simulink model "Trofazni_mosni_punoupravljivi_tiristorski_ispravljac"  (R2014b)
settings: Solver=ode5  StartTime=0.0  StopTime=1  FixedStep=Tsim  MaxStep=Tsim  RelTol=1e-3
values from neighbouring files (symbols this model uses):
  alfa = 60    [ParametriMfajl.m]
  f = 50    [ParametriMfajl.m]
  L = 10e-3    (= 0.01)    [ParametriMfajl.m]
  R = 10    [ParametriMfajl.m]
  Vmax = 220*sqrt(2)    [ParametriMfajl.m]
libraries: powerlib x20, powerlib_meascontrol x1
settings Model: Creator=Korisnik  LastModifiedBy=Zorana

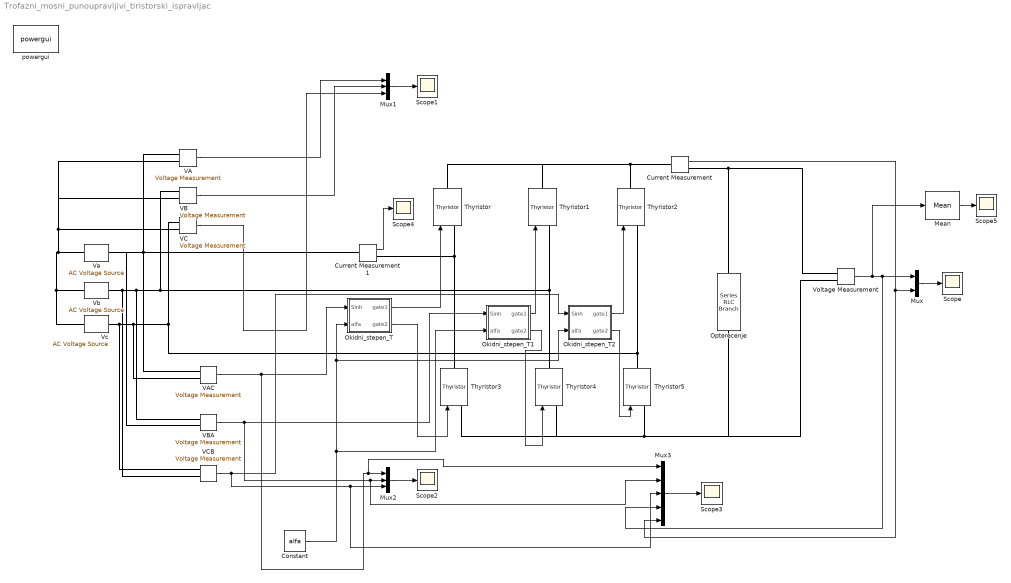
== system Trofazni_mosni_punoupravljivi_tiristorski_ispravljac ==
  Constant : Constant  Value=alfa
  Current Measurement : powerlib/Measurements/Current Measurement  PhasorSimulation=off  OutputType=Complex  PSBequivalent=0
  Current Measurement1 : powerlib/Measurements/Current Measurement  PhasorSimulation=off  OutputType=Complex  PSBequivalent=0
  Mean : powerlib_meascontrol/Measurements/Mean  Freq=f  Vinit=0  Ts=0
  Mux : Mux  Inputs=2
  Mux1 : Mux  Inputs=3
  Mux2 : Mux  Inputs=3
  Mux3 : Mux  Inputs=5
  Okidni_stepen_T : Subsystem
  Okidni_stepen_T1 : Subsystem
  Okidni_stepen_T2 : Subsystem
  Opterecenje : powerlib/Elements/Series RLC Branch  LConnTagsString=__new0  RConnTagsString=__new0  BranchType=RL  Resistance=R  Inductance=L*100  SetiL0=off  InitialCurrent=0  Capacitance=1e-6  Setx0=off  InitialVoltage=0  Measurements=None
  Scope{,1..5} (6 alike) : Scope
      Scope settings: YMin=-300  YMax=300
      Scope2 settings: SaveName=ScopeData2
      Scope3 settings: SaveName=ScopeData3
      Scope4 settings: SaveName=ScopeData4
      Scope5 settings: YMin=-300  YMax=300  SaveName=ScopeData5
  Thyristor{,1..5} (6 alike) : powerlib/Power Electronics/Thyristor  Ron=1e-6  Lon=0  Vf=0  IC=0  Rs=500  Cs=250e-9  Measurements=off
  VA : powerlib/Measurements/Voltage Measurement  PhasorSimulation=off  OutputType=Complex  PSBequivalent=0
  VAC : powerlib/Measurements/Voltage Measurement  PhasorSimulation=off  OutputType=Complex  PSBequivalent=0
  VB : powerlib/Measurements/Voltage Measurement  PhasorSimulation=off  OutputType=Complex  PSBequivalent=0
  VBA : powerlib/Measurements/Voltage Measurement  PhasorSimulation=off  OutputType=Complex  PSBequivalent=0
  VC : powerlib/Measurements/Voltage Measurement  PhasorSimulation=off  OutputType=Complex  PSBequivalent=0
  VCB : powerlib/Measurements/Voltage Measurement  PhasorSimulation=off  OutputType=Complex  PSBequivalent=0
  Va : powerlib/Electrical Sources/AC Voltage Source  Amplitude=Vmax  Phase=0  Frequency=f  SampleTime=0  Measurements=None
  Vb : powerlib/Electrical Sources/AC Voltage Source  Amplitude=Vmax  Phase=-120  Frequency=f  SampleTime=0  Measurements=None
  Vc : powerlib/Electrical Sources/AC Voltage Source  Amplitude=Vmax  Phase=-240  Frequency=f  SampleTime=0  Measurements=None
  Voltage Measurement : powerlib/Measurements/Voltage Measurement  PhasorSimulation=off  OutputType=Complex  PSBequivalent=0
  powergui : powerlib/powergui  Priority=1  SimulationMode=Continuous  SolverType=Tustin/Backward Euler (TBE)  SampleTime=50e-6  frequency=60  SPID=off  DisableSnubberDevices=off  DisableRonSwitches=off  DisableVfSwitches=off  SwTol=0  DisplayEquations=off  Interpol=off  methode=off  Ts=100  frequencyindice=50  Pbase=100e6  ErrMax=1e-4  Iterations=50  UnitsV=kV  UnitsW=MW  FunctionMessages=off  echomessages=off  HookPort=off  EnableUseOfTLC=off  x0status=blocks  RestoreLinks=warning  ResistiveCurrentMeasurement=off  Frange=[0:2:500]  Ylog=off  Xlog=on  ShowGrid=off  save=off  variable=ZData  structure=0  ZoomFFT=off  StartTime=0.0  cycles=1  DisplayStyle=1  fundamental=60  FreqAxis=off  MaxFrequency=1000  frequencyindicesteady=1  RmsSteady=1  display=off
  wires:
  Voltage Measurement/1 -> Mean/1, Mux/1, Mux3/4
  Mux/1 -> Scope/1
  Mux1/1 -> Scope1/1
  VA/1 -> Mux1/1
  VB/1 -> Mux1/2
  VC/1 -> Mux1/3
  Mux2/1 -> Scope2/1
  Current Measurement/1 -> Mux3/5, Mux/2
  Mux3/1 -> Scope3/1
  Current Measurement1/1 -> Scope4/1
  Mean/1 -> Scope5/1
  VAC/1 -> Mux3/1, Mux2/1, Okidni_stepen_T/1(Sinh)
  Okidni_stepen_T/1(gate1) -> Thyristor/1
  Okidni_stepen_T/2(gate2) -> Thyristor3/1
  Constant/1 -> Okidni_stepen_T2/2(alfa), Okidni_stepen_T/2(alfa), Okidni_stepen_T1/2(alfa)
  VBA/1 -> Mux3/2, Mux2/2, Okidni_stepen_T1/1(Sinh)
  Okidni_stepen_T1/1(gate1) -> Thyristor1/1
  Okidni_stepen_T1/2(gate2) -> Thyristor4/1
  VCB/1 -> Mux3/3, Mux2/3, Okidni_stepen_T2/1(Sinh)
  Okidni_stepen_T2/1(gate1) -> Thyristor2/1
  Okidni_stepen_T2/2(gate2) -> Thyristor5/1
  connections:
  Current Measurement1/RConn1 -- Thyristor/LConn1 -- Thyristor3/RConn1
  Vb/RConn1 -- VCB/LConn2 -- VBA/LConn1 -- VB/LConn1 -- Thyristor1/LConn1 -- Thyristor4/RConn1
  Vc/RConn1 -- VCB/LConn1 -- VAC/LConn2 -- VC/LConn1 -- Thyristor2/LConn1 -- Thyristor5/RConn1
  Thyristor3/LConn1 -- Thyristor4/LConn1 -- Opterecenje/RConn1 -- Voltage Measurement/LConn2 -- Thyristor5/LConn1
  Current Measurement/LConn1 -- Thyristor/RConn1 -- Thyristor1/RConn1 -- Thyristor2/RConn1
  Current Measurement/RConn1 -- Voltage Measurement/LConn1 -- Opterecenje/LConn1
  Va/LConn1 -- VB/LConn2 -- VA/LConn2 -- VC/LConn2 -- Vb/LConn1 -- Vc/LConn1
  VA/LConn1 -- VBA/LConn2 -- Va/RConn1 -- VAC/LConn1 -- Current Measurement1/LConn1

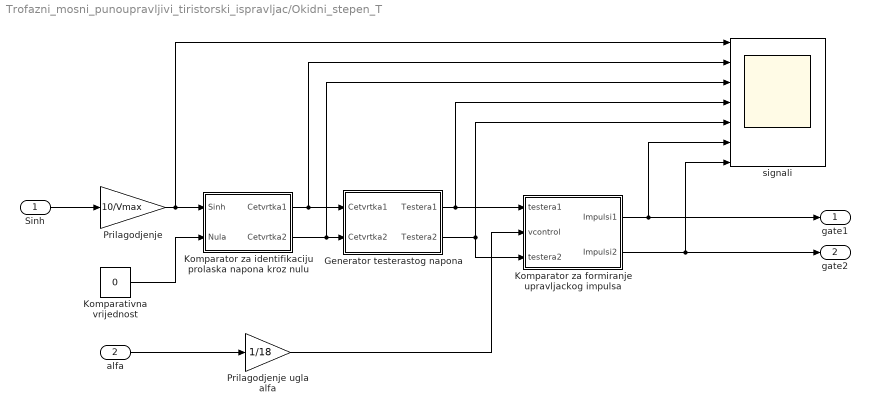
== system Trofazni_mosni_punoupravljivi_tiristorski_ispravljac/Okidni_stepen_T ==
  Sinh : Inport
  alfa : Inport  Port=2
  Generator testerastog napona : Subsystem
  Komparativna vrijednost : Constant  Value=0
  Komparator za formiranje upravljackog impulsa : Subsystem
  Komparator za identifikaciju prolaska napona kroz nulu : Subsystem
  Prilagodjenje : Gain  Gain=10/Vmax
  Prilagodjenje ugla alfa : Gain  Gain=1/18
  signali : Scope  NumInputPorts=7
      settings: YMin=-10~0~0~0~-5~-5~-5  YMax=10~10~10~10~5~5~5  SaveName=ScopeData3
  gate1 : Outport
  gate2 : Outport  Port=2
  wires:
  Komparator za formiranje upravljackog impulsa/1(Impulsi1) -> signali/6, gate1/1
  Komparator za identifikaciju prolaska napona kroz nulu/1(Cetvrtka1) -> signali/2, Generator testerastog napona/1(Cetvrtka1)
  Sinh/1 -> Prilagodjenje/1
  Prilagodjenje ugla alfa/1 -> Komparator za formiranje upravljackog impulsa/2(vcontrol)
  Prilagodjenje/1 -> signali/1, Komparator za identifikaciju prolaska napona kroz nulu/1(Sinh)
  Generator testerastog napona/1(Testera1) -> signali/4, Komparator za formiranje upravljackog impulsa/1(testera1)
  alfa/1 -> Prilagodjenje ugla alfa/1
  Komparativna vrijednost/1 -> Komparator za identifikaciju prolaska napona kroz nulu/2(Nula)
  Komparator za identifikaciju prolaska napona kroz nulu/2(Cetvrtka2) -> signali/3, Generator testerastog napona/2(Cetvrtka2)
  Generator testerastog napona/2(Testera2) -> Komparator za formiranje upravljackog impulsa/3(testera2), signali/5
  Komparator za formiranje upravljackog impulsa/2(Impulsi2) -> signali/7, gate2/1

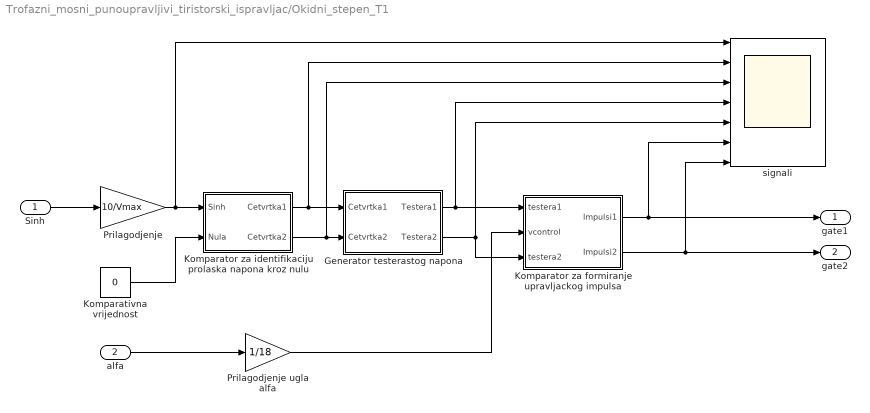
== system Trofazni_mosni_punoupravljivi_tiristorski_ispravljac/Okidni_stepen_T1 ==
  Sinh : Inport
  alfa : Inport  Port=2
  Generator testerastog napona : Subsystem
  Komparativna vrijednost : Constant  Value=0
  Komparator za formiranje upravljackog impulsa : Subsystem
  Komparator za identifikaciju prolaska napona kroz nulu : Subsystem
  Prilagodjenje : Gain  Gain=10/Vmax
  Prilagodjenje ugla alfa : Gain  Gain=1/18
  signali : Scope  NumInputPorts=7
      settings: YMin=-10~0~0~0~-5~-5~-5  YMax=10~10~10~10~5~5~5  SaveName=ScopeData3
  gate1 : Outport
  gate2 : Outport  Port=2
  wires:
  Komparator za formiranje upravljackog impulsa/2(Impulsi2) -> gate2/1, signali/7
  Generator testerastog napona/2(Testera2) -> signali/5, Komparator za formiranje upravljackog impulsa/3(testera2)
  Komparator za identifikaciju prolaska napona kroz nulu/2(Cetvrtka2) -> Generator testerastog napona/2(Cetvrtka2), signali/3
  Komparativna vrijednost/1 -> Komparator za identifikaciju prolaska napona kroz nulu/2(Nula)
  alfa/1 -> Prilagodjenje ugla alfa/1
  Generator testerastog napona/1(Testera1) -> Komparator za formiranje upravljackog impulsa/1(testera1), signali/4
  Prilagodjenje/1 -> Komparator za identifikaciju prolaska napona kroz nulu/1(Sinh), signali/1
  Prilagodjenje ugla alfa/1 -> Komparator za formiranje upravljackog impulsa/2(vcontrol)
  Sinh/1 -> Prilagodjenje/1
  Komparator za identifikaciju prolaska napona kroz nulu/1(Cetvrtka1) -> Generator testerastog napona/1(Cetvrtka1), signali/2
  Komparator za formiranje upravljackog impulsa/1(Impulsi1) -> gate1/1, signali/6

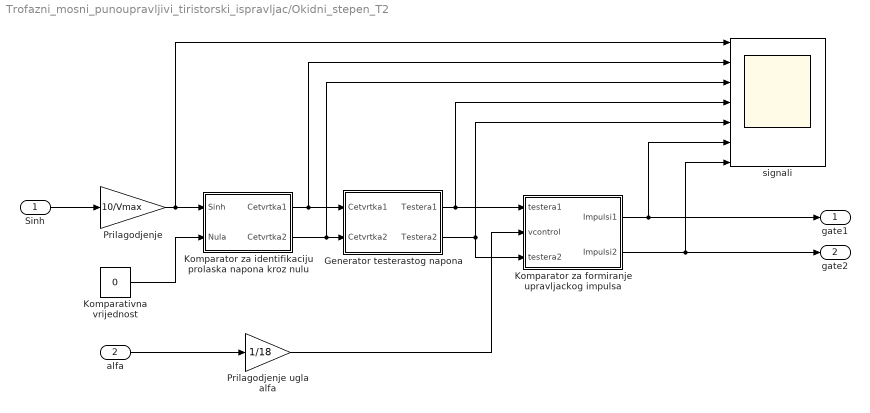
== system Trofazni_mosni_punoupravljivi_tiristorski_ispravljac/Okidni_stepen_T2 ==
  Sinh : Inport
  alfa : Inport  Port=2
  Generator testerastog napona : Subsystem
  Komparativna vrijednost : Constant  Value=0
  Komparator za formiranje upravljackog impulsa : Subsystem
  Komparator za identifikaciju prolaska napona kroz nulu : Subsystem
  Prilagodjenje : Gain  Gain=10/Vmax
  Prilagodjenje ugla alfa : Gain  Gain=1/18
  signali : Scope  NumInputPorts=7
      settings: YMin=-10~0~0~0~-5~-5~-5  YMax=10~10~10~10~5~5~5  SaveName=ScopeData3
  gate1 : Outport
  gate2 : Outport  Port=2
  wires:
  Komparator za formiranje upravljackog impulsa/1(Impulsi1) -> signali/6, gate1/1
  Komparator za identifikaciju prolaska napona kroz nulu/1(Cetvrtka1) -> signali/2, Generator testerastog napona/1(Cetvrtka1)
  Sinh/1 -> Prilagodjenje/1
  Prilagodjenje ugla alfa/1 -> Komparator za formiranje upravljackog impulsa/2(vcontrol)
  Prilagodjenje/1 -> signali/1, Komparator za identifikaciju prolaska napona kroz nulu/1(Sinh)
  Generator testerastog napona/1(Testera1) -> signali/4, Komparator za formiranje upravljackog impulsa/1(testera1)
  alfa/1 -> Prilagodjenje ugla alfa/1
  Komparativna vrijednost/1 -> Komparator za identifikaciju prolaska napona kroz nulu/2(Nula)
  Komparator za identifikaciju prolaska napona kroz nulu/2(Cetvrtka2) -> signali/3, Generator testerastog napona/2(Cetvrtka2)
  Generator testerastog napona/2(Testera2) -> Komparator za formiranje upravljackog impulsa/3(testera2), signali/5
  Komparator za formiranje upravljackog impulsa/2(Impulsi2) -> signali/7, gate2/1

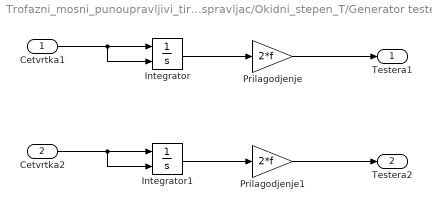
== system Trofazni_mosni_punoupravljivi_tiristorski_ispravljac/Okidni_stepen_T/Generator testerastog napona ==
  Cetvrtka1 : Inport
  Cetvrtka2 : Inport  Port=2
  Integrator : Integrator  ExternalReset=either
  Integrator1 : Integrator  ExternalReset=either
  Prilagodjenje : Gain  Gain=2*f
  Prilagodjenje1 : Gain  Gain=2*f
  Testera1 : Outport
  Testera2 : Outport  Port=2
  wires:
  Integrator/1 -> Prilagodjenje/1
  Cetvrtka1/1 -> Integrator/1, Integrator/2
  Prilagodjenje/1 -> Testera1/1
  Integrator1/1 -> Prilagodjenje1/1
  Cetvrtka2/1 -> Integrator1/2, Integrator1/1
  Prilagodjenje1/1 -> Testera2/1

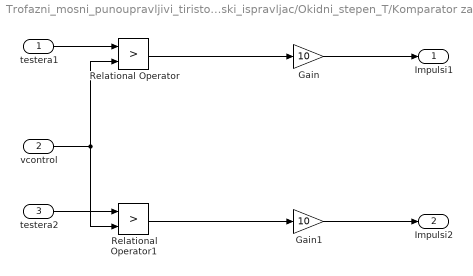
== system Trofazni_mosni_punoupravljivi_tiristorski_ispravljac/Okidni_stepen_T/Komparator za formiranje upravljackog impulsa ==
  testera1 : Inport
  vcontrol : Inport  Port=2
  testera2 : Inport  Port=3
  Gain : Gain  Gain=10
  Gain1 : Gain  Gain=10
  Relational Operator : RelationalOperator  Operator=>  OutDataTypeStr=fixdt(1,16)  InputSameDT=on
  Relational Operator1 : RelationalOperator  Operator=>  OutDataTypeStr=fixdt(1,16)  InputSameDT=on
  Impulsi1 : Outport
  Impulsi2 : Outport  Port=2
  wires:
  vcontrol/1 -> Relational Operator/2, Relational Operator1/2
  testera1/1 -> Relational Operator/1
  Gain/1 -> Impulsi1/1
  testera2/1 -> Relational Operator1/1
  Gain1/1 -> Impulsi2/1
  Relational Operator/1 -> Gain/1
  Relational Operator1/1 -> Gain1/1

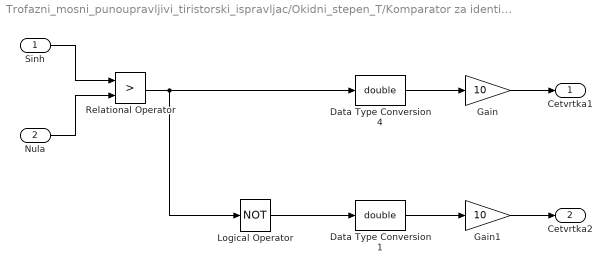
== system Trofazni_mosni_punoupravljivi_tiristorski_ispravljac/Okidni_stepen_T/Komparator za identifikaciju prolaska napona kroz nulu ==
  Sinh : Inport
  Nula : Inport  Port=2
  Data Type Conversion1 : DataTypeConversion  OutDataTypeStr=double  SaturateOnIntegerOverflow=on  RndMeth=Zero
  Data Type Conversion4 : DataTypeConversion  OutDataTypeStr=double  SaturateOnIntegerOverflow=on  RndMeth=Zero
  Gain : Gain  Gain=10
  Gain1 : Gain  Gain=10
  Logical Operator : Logic  Operator=NOT  IconShape=distinctive  AllPortsSameDT=off  OutDataTypeStr=boolean
  Relational Operator : RelationalOperator  Operator=>  OutDataTypeStr=fixdt(1,16)  InputSameDT=on
  Cetvrtka1 : Outport
  Cetvrtka2 : Outport  Port=2
  wires:
  Gain/1 -> Cetvrtka1/1
  Sinh/1 -> Relational Operator/1
  Nula/1 -> Relational Operator/2
  Relational Operator/1 -> Logical Operator/1, Data Type Conversion4/1
  Data Type Conversion4/1 -> Gain/1
  Gain1/1 -> Cetvrtka2/1
  Data Type Conversion1/1 -> Gain1/1
  Logical Operator/1 -> Data Type Conversion1/1

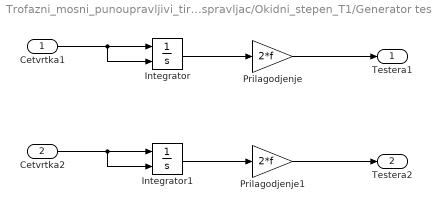
== system Trofazni_mosni_punoupravljivi_tiristorski_ispravljac/Okidni_stepen_T1/Generator testerastog napona ==
  Cetvrtka1 : Inport
  Cetvrtka2 : Inport  Port=2
  Integrator : Integrator  ExternalReset=either
  Integrator1 : Integrator  ExternalReset=either
  Prilagodjenje : Gain  Gain=2*f
  Prilagodjenje1 : Gain  Gain=2*f
  Testera1 : Outport
  Testera2 : Outport  Port=2
  wires:
  Prilagodjenje1/1 -> Testera2/1
  Cetvrtka2/1 -> Integrator1/1, Integrator1/2
  Integrator1/1 -> Prilagodjenje1/1
  Prilagodjenje/1 -> Testera1/1
  Cetvrtka1/1 -> Integrator/2, Integrator/1
  Integrator/1 -> Prilagodjenje/1

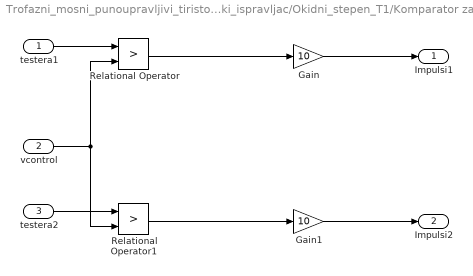
== system Trofazni_mosni_punoupravljivi_tiristorski_ispravljac/Okidni_stepen_T1/Komparator za formiranje upravljackog impulsa ==
  testera1 : Inport
  vcontrol : Inport  Port=2
  testera2 : Inport  Port=3
  Gain : Gain  Gain=10
  Gain1 : Gain  Gain=10
  Relational Operator : RelationalOperator  Operator=>  OutDataTypeStr=fixdt(1,16)  InputSameDT=on
  Relational Operator1 : RelationalOperator  Operator=>  OutDataTypeStr=fixdt(1,16)  InputSameDT=on
  Impulsi1 : Outport
  Impulsi2 : Outport  Port=2
  wires:
  Relational Operator1/1 -> Gain1/1
  Relational Operator/1 -> Gain/1
  Gain1/1 -> Impulsi2/1
  testera2/1 -> Relational Operator1/1
  Gain/1 -> Impulsi1/1
  testera1/1 -> Relational Operator/1
  vcontrol/1 -> Relational Operator1/2, Relational Operator/2

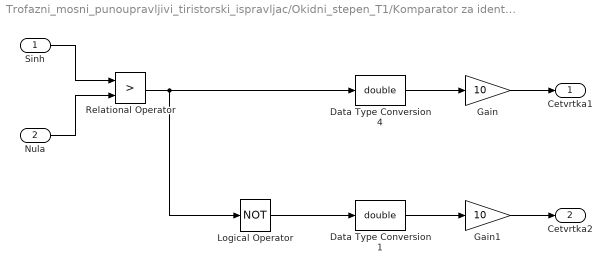
== system Trofazni_mosni_punoupravljivi_tiristorski_ispravljac/Okidni_stepen_T1/Komparator za identifikaciju prolaska napona kroz nulu ==
  Sinh : Inport
  Nula : Inport  Port=2
  Data Type Conversion1 : DataTypeConversion  OutDataTypeStr=double  SaturateOnIntegerOverflow=on  RndMeth=Zero
  Data Type Conversion4 : DataTypeConversion  OutDataTypeStr=double  SaturateOnIntegerOverflow=on  RndMeth=Zero
  Gain : Gain  Gain=10
  Gain1 : Gain  Gain=10
  Logical Operator : Logic  Operator=NOT  IconShape=distinctive  AllPortsSameDT=off  OutDataTypeStr=boolean
  Relational Operator : RelationalOperator  Operator=>  OutDataTypeStr=fixdt(1,16)  InputSameDT=on
  Cetvrtka1 : Outport
  Cetvrtka2 : Outport  Port=2
  wires:
  Logical Operator/1 -> Data Type Conversion1/1
  Data Type Conversion1/1 -> Gain1/1
  Gain1/1 -> Cetvrtka2/1
  Data Type Conversion4/1 -> Gain/1
  Relational Operator/1 -> Data Type Conversion4/1, Logical Operator/1
  Nula/1 -> Relational Operator/2
  Sinh/1 -> Relational Operator/1
  Gain/1 -> Cetvrtka1/1

== system Trofazni_mosni_punoupravljivi_tiristorski_ispravljac/Okidni_stepen_T2/Generator testerastog napona ==
  Cetvrtka1 : Inport
  Cetvrtka2 : Inport  Port=2
  Integrator : Integrator  ExternalReset=either
  Integrator1 : Integrator  ExternalReset=either
  Prilagodjenje : Gain  Gain=2*f
  Prilagodjenje1 : Gain  Gain=2*f
  Testera1 : Outport
  Testera2 : Outport  Port=2
  wires:
  Integrator/1 -> Prilagodjenje/1
  Cetvrtka1/1 -> Integrator/1, Integrator/2
  Prilagodjenje/1 -> Testera1/1
  Integrator1/1 -> Prilagodjenje1/1
  Cetvrtka2/1 -> Integrator1/2, Integrator1/1
  Prilagodjenje1/1 -> Testera2/1

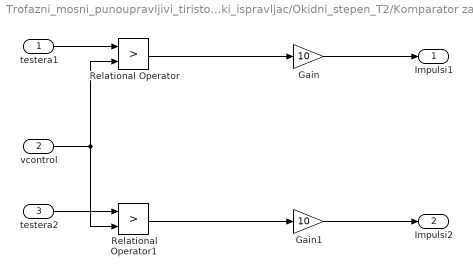
== system Trofazni_mosni_punoupravljivi_tiristorski_ispravljac/Okidni_stepen_T2/Komparator za formiranje upravljackog impulsa ==
  testera1 : Inport
  vcontrol : Inport  Port=2
  testera2 : Inport  Port=3
  Gain : Gain  Gain=10
  Gain1 : Gain  Gain=10
  Relational Operator : RelationalOperator  Operator=>  OutDataTypeStr=fixdt(1,16)  InputSameDT=on
  Relational Operator1 : RelationalOperator  Operator=>  OutDataTypeStr=fixdt(1,16)  InputSameDT=on
  Impulsi1 : Outport
  Impulsi2 : Outport  Port=2
  wires:
  vcontrol/1 -> Relational Operator/2, Relational Operator1/2
  testera1/1 -> Relational Operator/1
  Gain/1 -> Impulsi1/1
  testera2/1 -> Relational Operator1/1
  Gain1/1 -> Impulsi2/1
  Relational Operator/1 -> Gain/1
  Relational Operator1/1 -> Gain1/1

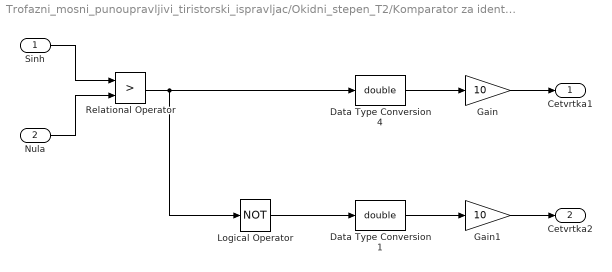
== system Trofazni_mosni_punoupravljivi_tiristorski_ispravljac/Okidni_stepen_T2/Komparator za identifikaciju prolaska napona kroz nulu ==
  Sinh : Inport
  Nula : Inport  Port=2
  Data Type Conversion1 : DataTypeConversion  OutDataTypeStr=double  SaturateOnIntegerOverflow=on  RndMeth=Zero
  Data Type Conversion4 : DataTypeConversion  OutDataTypeStr=double  SaturateOnIntegerOverflow=on  RndMeth=Zero
  Gain : Gain  Gain=10
  Gain1 : Gain  Gain=10
  Logical Operator : Logic  Operator=NOT  IconShape=distinctive  AllPortsSameDT=off  OutDataTypeStr=boolean
  Relational Operator : RelationalOperator  Operator=>  OutDataTypeStr=fixdt(1,16)  InputSameDT=on
  Cetvrtka1 : Outport
  Cetvrtka2 : Outport  Port=2
  wires:
  Gain/1 -> Cetvrtka1/1
  Sinh/1 -> Relational Operator/1
  Nula/1 -> Relational Operator/2
  Relational Operator/1 -> Logical Operator/1, Data Type Conversion4/1
  Data Type Conversion4/1 -> Gain/1
  Gain1/1 -> Cetvrtka2/1
  Data Type Conversion1/1 -> Gain1/1
  Logical Operator/1 -> Data Type Conversion1/1
